simulink model "Aerosonde_sim"  (R2017a)
settings: Solver=VariableStepAuto  StartTime=0.0  StopTime=600.0  RelTol=1e-3
values from neighbouring files (symbols this model uses):
  b = 2.8956    [coeff.m]
  c = 0.18994    [coeff.m]
  C_De = 0    [coeff.m]
  C_Dq = 0    [coeff.m]
  C_Le = -0.36    [coeff.m]
  C_Lq = 0    [coeff.m]
  C_m0 = -0.02338    [coeff.m]
  C_ma = -0.38    [coeff.m]
  C_me = -0.5    [coeff.m]
  C_mq = -3.6    [coeff.m]
  rho = 1.2682    [coeff.m]
libraries: simulink_extras x2, aerolibasang x2, shared3dof x1, aerolibadyn x1
settings Model: Creator=jljoberg  LastModifiedBy=jljoberg

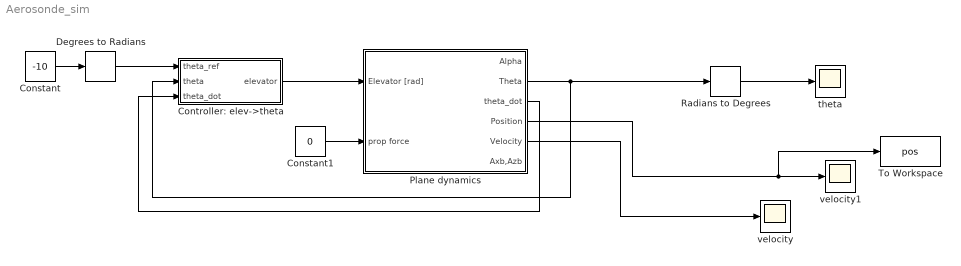
== system Aerosonde_sim ==
  Constant : Constant  Value=-10
  Constant1 : Constant  Value=0
  Controller: elev->theta : Subsystem
  Degrees to Radians : simulink_extras/Transformations/Degrees to Radians
  Plane dynamics : Subsystem
  Radians to Degrees : simulink_extras/Transformations/Radians to Degrees
  To Workspace : ToWorkspace  VariableName=pos  SaveFormat=Timeseries  SampleTime=-1
  theta : Scope
  velocity : Scope
  velocity1 : Scope
  wires:
  Controller: elev->theta/1(elevator) -> Plane dynamics/1(Elevator [rad])
  Constant/1 -> Degrees to Radians/1
  Constant1/1 -> Plane dynamics/2(prop force)
  Plane dynamics/2(Theta) -> Controller: elev->theta/2(theta), Radians to Degrees/1
  Degrees to Radians/1 -> Controller: elev->theta/1(theta_ref)
  Plane dynamics/3(theta_dot) -> Controller: elev->theta/3(theta_dot)
  Radians to Degrees/1 -> theta/1
  Plane dynamics/5(Velocity) -> velocity/1
  Plane dynamics/4(Position) -> To Workspace/1, velocity1/1

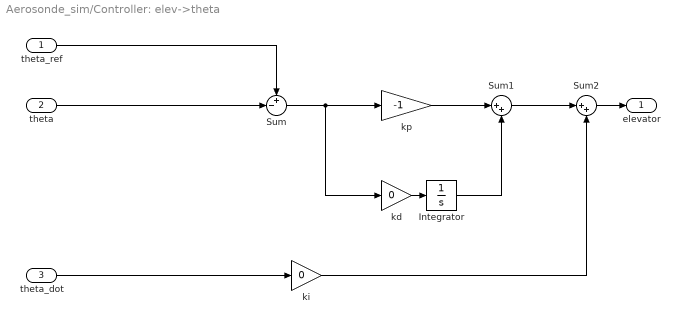
== system Aerosonde_sim/Controller: elev->theta ==
  theta_ref : Inport
  theta : Inport  Port=2
  theta_dot : Inport  Port=3
  Integrator : Integrator
  Sum : Sum  Inputs=+-|
  Sum1 : Sum  Inputs=|++
  Sum2 : Sum  Inputs=|++
  kd : Gain  Gain=0
  ki : Gain  Gain=0
  kp : Gain  Gain=-1
  elevator : Outport
  wires:
  theta/1 -> Sum/2
  theta_ref/1 -> Sum/1
  Sum/1 -> kd/1, kp/1
  kp/1 -> Sum1/1
  kd/1 -> Integrator/1
  Integrator/1 -> Sum1/2
  Sum1/1 -> Sum2/1
  Sum2/1 -> elevator/1
  theta_dot/1 -> ki/1
  ki/1 -> Sum2/2

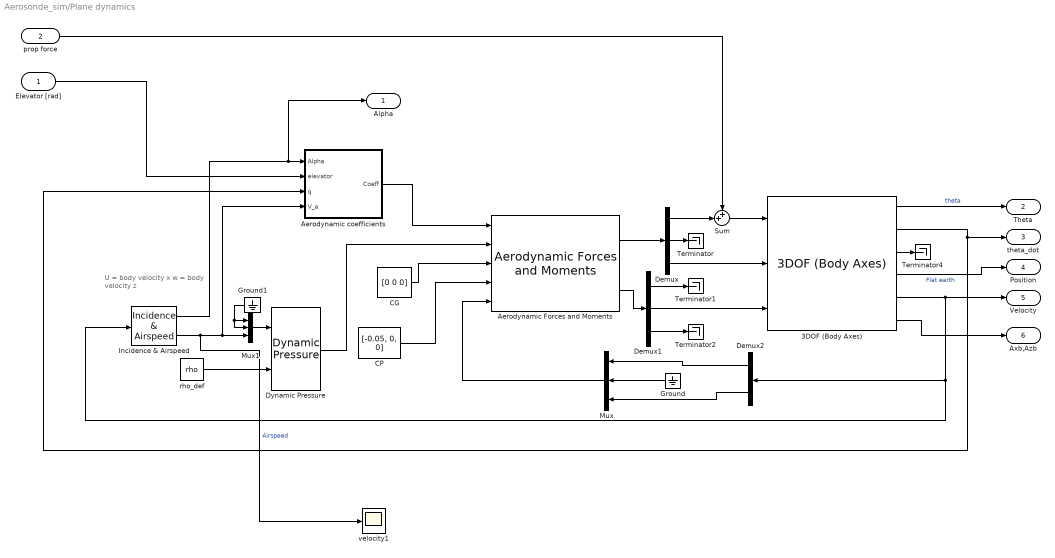
== system Aerosonde_sim/Plane dynamics ==
  note: U = body velocity x
      | w = body velocity z
  Elevator [rad] : Inport
  prop force : Inport  Port=2
  3DOF (Body Axes) : shared3dof/3DOF (Body Axes)  units=Metric (MKS)  mtype=Fixed  v_ini=20  theta_ini=0  alpha_ini=0  q_ini=0  pos_ini=[0 0]  mass=m  mass_e=0.5  mass_f=3.0  Iyy=Jy  Iyy_e=0.5  Iyy_f=3.0  g_in=Internal  g=9.81  vre_flag=on  abi_flag=off
  "Aerodynamic Forces and Moments " : aerolibadyn/Aerodynamic Forces and Moments   inputAxes=Wind  outputForceAxes=Body  outputMomentAxes=Wind  S=S  b=b  cbar=1
      settings: SourceProductName=Aerospace Blockset
  Aerodynamic coefficients : Subsystem
  CG : Constant  Value=[0 0 0]
  CP : Constant  Value=[-0.05, 0, 0]
  Demux : Demux  Outputs=3
  Demux1 : Demux  Outputs=3
  Demux2 : Demux  Outputs=2
  Dynamic Pressure : aerolibasang/Dynamic Pressure
  Ground : Ground
  Ground1 : Ground
  Incidence & Airspeed : aerolibasang/Incidence  & Airspeed
      settings: SourceProductName=Aerospace Blockset  SourceProductBaseCode=AE
  Mux : Mux  Inputs=3
  Mux1 : Mux  Inputs=3
  Sum : Sum  Inputs=++|
  Terminator{,1..2,4} (4 alike) : Terminator
  rho_def : Constant  Value=rho
  velocity1 : Scope
  Alpha : Outport
  Theta : Outport  Port=2
  theta_dot : Outport  Port=3
  Position : Outport  Port=4
  Velocity : Outport  Port=5
  Axb,Azb : Outport  Port=6
  wires:
  Ground1/1 -> Mux1/1, Mux1/2
  3DOF (Body Axes)/2 -> theta_dot/1, Aerodynamic coefficients/3(q)
  3DOF (Body Axes)/3 -> Terminator4/1
  Incidence & Airspeed/1 -> Alpha/1, Aerodynamic coefficients/1(Alpha)
  "Aerodynamic Forces and Moments "/1 -> Demux/1
  rho_def/1 -> Dynamic Pressure/2
  Aerodynamic coefficients/1(Coeff) -> "Aerodynamic Forces and Moments "/1
  Incidence & Airspeed/2 -> velocity1/1, Mux1/3, Aerodynamic coefficients/4(V_a)  "Airspeed"
  3DOF (Body Axes)/5 -> Velocity/1, Demux2/1, Incidence & Airspeed/1
  Dynamic Pressure/1 -> "Aerodynamic Forces and Moments "/2
  Demux/3 -> 3DOF (Body Axes)/2
  "Aerodynamic Forces and Moments "/2 -> Demux1/1
  3DOF (Body Axes)/1 -> Theta/1  "theta"
  3DOF (Body Axes)/6 -> Axb,Azb/1
  Demux/2 -> Terminator/1
  3DOF (Body Axes)/4 -> Position/1  "Flat earth"
  CG/1 -> "Aerodynamic Forces and Moments "/3
  CP/1 -> "Aerodynamic Forces and Moments "/4
  Demux2/1 -> Mux/1
  Demux1/2 -> 3DOF (Body Axes)/3
  Ground/1 -> Mux/2
  Demux1/1 -> Terminator1/1
  Demux1/3 -> Terminator2/1
  Demux2/2 -> Mux/3
  Mux/1 -> "Aerodynamic Forces and Moments "/5
  Elevator [rad]/1 -> Aerodynamic coefficients/2(elevator)
  Mux1/1 -> Dynamic Pressure/1
  Sum/1 -> 3DOF (Body Axes)/1
  prop force/1 -> Sum/1
  Demux/1 -> Sum/2

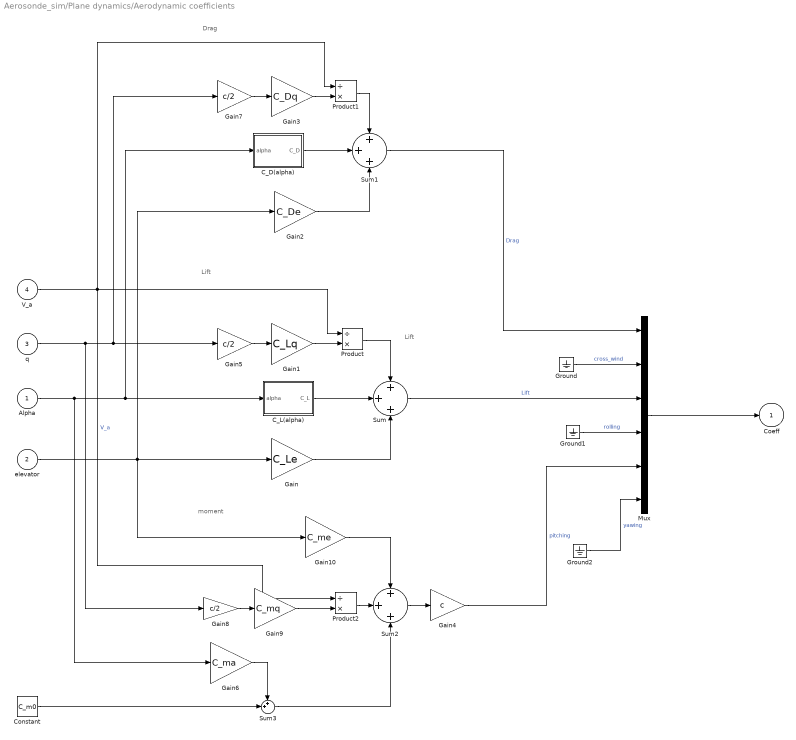
== system Aerosonde_sim/Plane dynamics/Aerodynamic coefficients ==
  note: moment
  note: Lift
  note: Drag
  note: Lift
  Alpha : Inport
  elevator : Inport  Port=2
  q : Inport  Port=3
  V_a : Inport  Port=4
  C_D(alpha) : MATLAB Function  TreatAsAtomicUnit=on
  C_L(alpha) : MATLAB Function  TreatAsAtomicUnit=on
  Constant : Constant  Value=C_m0
  Gain : Gain  Gain=C_Le
  Gain1 : Gain  Gain=C_Lq
  Gain10 : Gain  Gain=C_me
  Gain2 : Gain  Gain=C_De
  Gain3 : Gain  Gain=C_Dq
  Gain4 : Gain  Gain=c
  Gain5 : Gain  Gain=c/2
  Gain6 : Gain  Gain=C_ma
  Gain7 : Gain  Gain=c/2
  Gain8 : Gain  Gain=c/2
  Gain9 : Gain  Gain=C_mq
  Ground : Ground
  Ground1 : Ground
  Ground2 : Ground
  Mux : Mux  Inputs=6
  Product : Product  Inputs=/*
  Product1 : Product  Inputs=/*
  Product2 : Product  Inputs=/*
  Sum : Sum  Inputs=+++
  Sum1 : Sum  Inputs=+++
  Sum2 : Sum  Inputs=+++
  Sum3 : Sum  Inputs=++|
  Coeff : Outport
  wires:
  Alpha/1 -> Gain6/1, C_D(alpha)/1(alpha), C_L(alpha)/1(alpha)
  C_L(alpha)/1(C_L) -> Sum/2
  Gain/1 -> Sum/3
  Sum/1 -> Mux/3  "Lift"
  Ground/1 -> Mux/2  "cross_wind"
  Ground1/1 -> Mux/4  "rolling"
  Ground2/1 -> Mux/6  "yawing"
  C_D(alpha)/1(C_D) -> Sum1/2
  Gain2/1 -> Sum1/3
  q/1 -> Gain8/1, Gain7/1, Gain5/1
  V_a/1 -> Product2/1, Product/1, Product1/1  "V_a"
  Gain1/1 -> Product/2
  Product/1 -> Sum/1
  Gain5/1 -> Gain1/1
  Gain3/1 -> Product1/2
  Product1/1 -> Sum1/1
  Gain7/1 -> Gain3/1
  Sum1/1 -> Mux/1  "Drag"
  Sum2/1 -> Gain4/1
  Gain4/1 -> Mux/5  "pitching"
  Constant/1 -> Sum3/2
  Sum3/1 -> Sum2/3
  Gain6/1 -> Sum3/1
  Product2/1 -> Sum2/2
  Gain8/1 -> Gain9/1
  Gain9/1 -> Product2/2
  Gain10/1 -> Sum2/1
  elevator/1 -> Gain10/1, Gain2/1, Gain/1
  Mux/1 -> Coeff/1

== matlab function Aerosonde_sim/Plane dynamics/Aerodynamic coefficients/C_D(alpha) ==
  data: alpha input; C_D output
function C_D = C_D(alpha)


C_Dp    = 0.0437; 
C_L0    = 0.28;
C_La    = 3.45;
e       = 0.9;
S       = 0.55;
b       = 2.8956;
AR      = b^2/S;

C_D = C_Dp + (C_L0 + C_La*alpha)^2/(pi*e*AR);

== matlab function Aerosonde_sim/Plane dynamics/Aerodynamic coefficients/C_L(alpha) ==
  data: alpha input; C_L output
function C_L = C_L(alpha)

C_L0    = 0.28; 
C_La    = 3.45;
M       = 50;

alpha_0 = 0.4712;
sigma =( 1+exp(-M*(alpha-alpha_0))+exp(M*(alpha+alpha_0)) ) ...
              / ( (1+exp(-M*(alpha-alpha_0)))*(1+exp(M*(alpha+alpha_0))) );


C_L = (1-sigma) * (C_L0 + C_La*alpha) ...
             + sigma * 2*sign(alpha)*sin(alpha)^2*cos(alpha);
